simulink model "example23"  (R2023b)
settings: Solver=VariableStepAuto  StartTime=0.0  StopTime=10.0  RelTol=1e-3
settings Model: Creator=ray  LastModifiedBy=ray

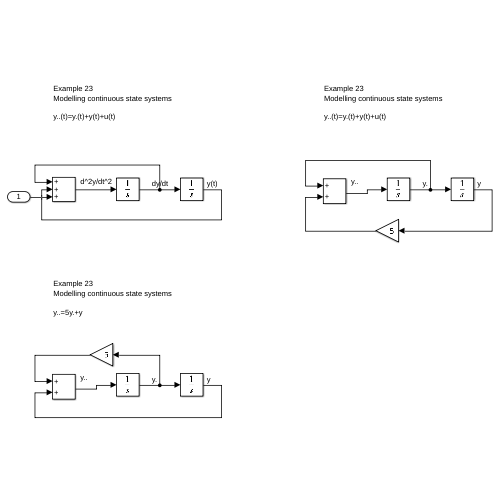
[thumbnail: Simulink's stored preview of the top-level diagram]
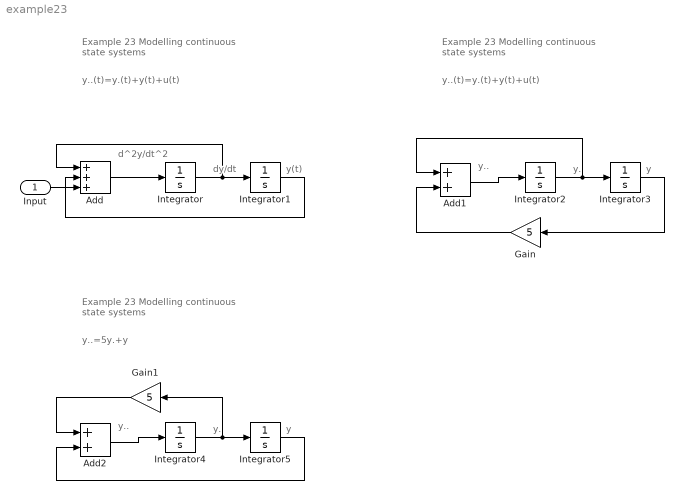
== system example23 ==
  note: y(t)
  note: y..(t)=y.(t)+y(t)+u(t)
  note: d^2y/dt^2
  note: dy/dt
  note: Example 23
      | Modelling continuous state systems
  note: y..
  note: Example 23
      | Modelling continuous state systems
  note: y.
  note: y
  note: y..(t)=y.(t)+y(t)+u(t)
  note: y
  note: Example 23
      | Modelling continuous state systems
  note: y..
  note: y.
  note: y..=5y.+y
  Input : Inport
  Add : Sum  Inputs=+++
  Add1 : Sum
  Add2 : Sum
  Gain : Gain  Gain=5
  Gain1 : Gain  Gain=5
  Integrator{,1..5} (6 alike) : Integrator
  wires:
  Add/1 -> Integrator/1
  Integrator/1 -> Add/1, Integrator1/1
  Input/1 -> Add/3
  Integrator1/1 -> Add/2
  Integrator3/1 -> Gain/1
  Add1/1 -> Integrator2/1
  Integrator2/1 -> Add1/1, Integrator3/1
  Gain/1 -> Add1/2
  Add2/1 -> Integrator4/1
  Integrator4/1 -> Gain1/1, Integrator5/1
  Gain1/1 -> Add2/1
  Integrator5/1 -> Add2/2
